simulink model "system_5"  (R2022b)
settings: Solver=VariableStepAuto  StartTime=0.0  StopTime=12  MaxStep=1e-4  RelTol=1e-3
settings Model: Creator=Dongr  LastModifiedBy=Dong

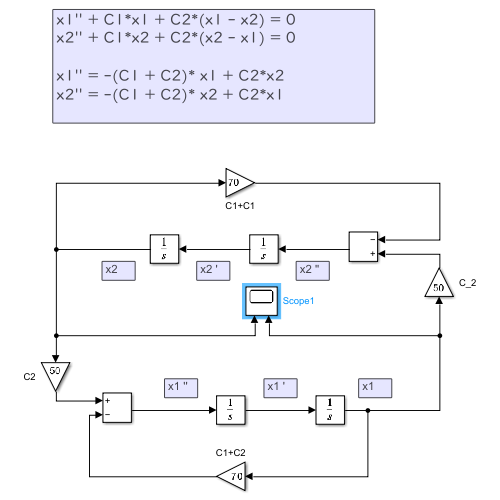
[thumbnail: Simulink's stored preview of the top-level diagram]
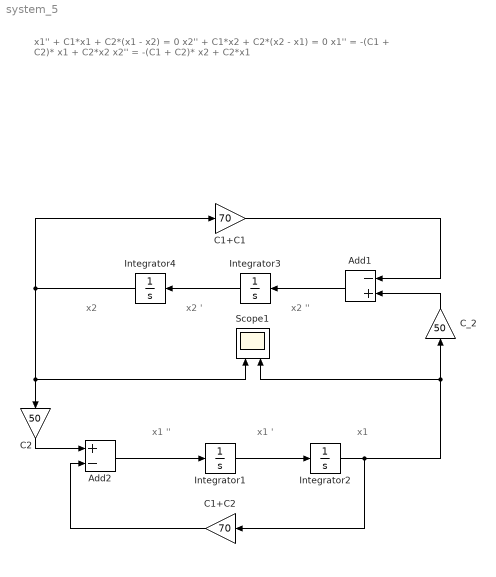
== system system_5 ==
  note: x1'' + C1*x1 + C2*(x1 - x2) = 0
      | x2'' + C1*x2 + C2*(x2 - x1) = 0
      |
      | x1'' = -(C1 + C2)* x1 + C2*x2
      | x2'' = -(C1 + C2)* x2 + C2*x1
  note: x1 ''
  note: x1 '
  note: x1
  note: x2 '
  note: x2
  note: x2 ''
  Add1 : Sum  Inputs=-+
  Add2 : Sum  Inputs=+-
  C1+C1 : Gain  Gain=70
  C1+C2 : Gain  Gain=70
  C2 : Gain  Gain=50
  C_2 : Gain  Gain=50
  Integrator1 : Integrator
  Integrator2 : Integrator  InitialCondition=0.5
  Integrator3 : Integrator
  Integrator4 : Integrator
  Scope1 : Scope  NumInputPorts=2
  wires:
  Integrator1/1 -> Integrator2/1
  Integrator3/1 -> Integrator4/1
  Add1/1 -> Integrator3/1
  Integrator4/1 -> C1+C1/1, Scope1/1, C2/1
  C2/1 -> Add2/1
  Add2/1 -> Integrator1/1
  C1+C2/1 -> Add2/2
  C_2/1 -> Add1/2
  C1+C1/1 -> Add1/1
  Integrator2/1 -> Scope1/2, C_2/1, C1+C2/1
